simulink model "Scenario_2_v2"  (R2020b)
settings: Solver=ode1  StartTime=0.0  StopTime=10  FixedStep=Ts  MaxStep=Ts*2  MinStep=Ts/5  RelTol=1e-3
values from neighbouring files (symbols this model uses):
  c0 = c0_zeb    (= 6.57988e-09)    [Scenario_17_parameters_v2.m]    (also in Scenario_1_parameters_v2.m; Scenario_2_parameters_v2.m; Scenario_3_parameters_v2.m)
  c1 = c1_zeb    (= 9.15905e-09)    [Scenario_17_parameters_v2.m]    (also in Scenario_1_parameters_v2.m; Scenario_2_parameters_v2.m; Scenario_3_parameters_v2.m)
  fg = 50    [Scenario_17_parameters_v2.m]    (also in Scenario_1_parameters_v2.m; Scenario_2_parameters_v2.m; Scenario_3_parameters_v2.m)
  G1gen = 0.4692    [Scenario_17_parameters_v2.m]    (also in Scenario_1_parameters_v2.m = 0.1; Scenario_2_parameters_v2.m = 0.298581; Scenario_3_parameters_v2.m = 0.65)
  G2gen = 0.80    (= 0.8)    [Scenario_1_parameters_v2.m]    (also in Scenario_2_parameters_v2.m = 0.7; Scenario_3_parameters_v2.m = 0.4)
  G3gen = 0.85    [Scenario_1_parameters_v2.m]    (also in Scenario_2_parameters_v2.m = 0.9; Scenario_3_parameters_v2.m = 0.6)
  G4sgen = 0.8186    [Scenario_2_parameters_v2.m]
  G5gen = 0.75    [Scenario_17_parameters_v2.m]    (also in Scenario_1_parameters_v2.m = 0.8; Scenario_2_parameters_v2.m = 0.8; Scenario_3_parameters_v2.m = 0.705)
  G6gen = 0.90    (= 0.9)    [Scenario_17_parameters_v2.m]    (also in Scenario_1_parameters_v2.m; Scenario_2_parameters_v2.m = 0.81797; Scenario_3_parameters_v2.m = 0.45)
  G6sgen = 0.7    [Scenario_2_parameters_v2.m]
  G7gen = 0.20    (= 0.2)    [Scenario_17_parameters_v2.m]    (also in Scenario_1_parameters_v2.m = 0.5227; Scenario_2_parameters_v2.m = 0.5098; Scenario_3_parameters_v2.m = 0.4)
  Iovc = 1.2    [Scenario_17_parameters_v2.m]    (also in Scenario_1_parameters_v2.m; Scenario_2_parameters_v2.m; Scenario_3_parameters_v2.m)
  l0 = l0_zeb    (= 0.00368)    [Scenario_17_parameters_v2.m]    (also in Scenario_1_parameters_v2.m; Scenario_2_parameters_v2.m; Scenario_3_parameters_v2.m)
  l1 = l1_zeb    (= 0.00128)    [Scenario_17_parameters_v2.m]    (also in Scenario_1_parameters_v2.m; Scenario_2_parameters_v2.m; Scenario_3_parameters_v2.m)
  L3dem = 0.30    (= 0.3)    [Scenario_17_parameters_v2.m]    (also in Scenario_1_parameters_v2.m = 0.1; Scenario_2_parameters_v2.m = 0.1; Scenario_3_parameters_v2.m = 0.2)
  L4dem = 0.30    (= 0.3)    [Scenario_1_parameters_v2.m]    (also in Scenario_2_parameters_v2.m)
  L5dem = 0.25    [Scenario_17_parameters_v2.m]    (also in Scenario_1_parameters_v2.m = 0.35; Scenario_2_parameters_v2.m = 0.35; Scenario_3_parameters_v2.m = 0.1)
  L6dem = 0.15    [Scenario_1_parameters_v2.m]    (also in Scenario_2_parameters_v2.m; Scenario_3_parameters_v2.m = 0.1)
  L7dem = 0.10    (= 0.1)    [Scenario_1_parameters_v2.m]    (also in Scenario_2_parameters_v2.m; Scenario_3_parameters_v2.m = 0.2)
  Pr = Sr*PF    (= 1600500000)    [Scenario_17_parameters_v2.m]    (also in Scenario_1_parameters_v2.m = 1472500000; Scenario_2_parameters_v2.m = 1805000000; Scenario_3_parameters_v2.m = 12740000000)
  Qr = sqrt(Sr^2 - Pr^2)    [Scenario_17_parameters_v2.m]    (also in Scenario_1_parameters_v2.m; Scenario_2_parameters_v2.m; Scenario_3_parameters_v2.m)
  r0 = r0_zeb    (= 0.39362)    [Scenario_17_parameters_v2.m]    (also in Scenario_1_parameters_v2.m; Scenario_2_parameters_v2.m; Scenario_3_parameters_v2.m)
  r1 = r1_zeb    (= 0.06862)    [Scenario_17_parameters_v2.m]    (also in Scenario_1_parameters_v2.m; Scenario_2_parameters_v2.m; Scenario_3_parameters_v2.m)
  Rtpu = Xtpu/40    (= 0.0025)    [Scenario_17_parameters_v2.m]    (also in Scenario_1_parameters_v2.m = 0.00375; Scenario_2_parameters_v2.m = 0.00375; Scenario_3_parameters_v2.m)
  S1non = 700e6    (= 700000000)    [Scenario_17_parameters_v2.m]    (also in Scenario_1_parameters_v2.m = 400000000; Scenario_2_parameters_v2.m = 400000000; Scenario_3_parameters_v2.m = 1000000000)
  S2non = 300e6    (= 300000000)    [Scenario_1_parameters_v2.m]    (also in Scenario_2_parameters_v2.m; Scenario_3_parameters_v2.m = 3000000000)
  S3non = 200e6    (= 200000000)    [Scenario_1_parameters_v2.m]    (also in Scenario_2_parameters_v2.m; Scenario_3_parameters_v2.m = 1000000000)
  S4snon = 200e6    (= 200000000)    [Scenario_2_parameters_v2.m]
  S5non = 400e6    (= 400000000)    [Scenario_17_parameters_v2.m]    (also in Scenario_1_parameters_v2.m = 500000000; Scenario_2_parameters_v2.m = 500000000; Scenario_3_parameters_v2.m = 2000000000)
  S6non = 150e6    (= 150000000)    [Scenario_17_parameters_v2.m]    (also in Scenario_1_parameters_v2.m = 400000000; Scenario_2_parameters_v2.m = 400000000; Scenario_3_parameters_v2.m = 3000000000)
  S6snon = 200e6    (= 200000000)    [Scenario_2_parameters_v2.m]
  S7non = 1500e6    (= 1500000000)    [Scenario_17_parameters_v2.m]    (also in Scenario_1_parameters_v2.m = 200000000; Scenario_2_parameters_v2.m = 200000000; Scenario_3_parameters_v2.m = 4000000000)
  tonvsc = 0    [Scenario_17_parameters_v2.m]    (also in Scenario_1_parameters_v2.m; Scenario_2_parameters_v2.m; Scenario_3_parameters_v2.m = 0.0001)
  Ts = 50e-6    (= 5e-05)    [Scenario_17_parameters_v2.m]    (also in Scenario_1_parameters_v2.m = 0.0002; Scenario_2_parameters_v2.m = 2e-05; Scenario_3_parameters_v2.m = 0.0001)
  Vhv = 220e3    (= 220000)    [Scenario_17_parameters_v2.m]    (also in Scenario_1_parameters_v2.m; Scenario_2_parameters_v2.m; Scenario_3_parameters_v2.m)
  Vmv = 22e3    (= 22000)    [Scenario_17_parameters_v2.m]    (also in Scenario_1_parameters_v2.m; Scenario_2_parameters_v2.m; Scenario_3_parameters_v2.m)
  w_pll = 2*pi*80    (= 502.654824574)    [Scenario_17_parameters_v2.m]    (also in Scenario_1_parameters_v2.m; Scenario_2_parameters_v2.m; Scenario_3_parameters_v2.m)
  wc1 = wsw1/10    (= 848.230016469)    [Scenario_17_parameters_v2.m]    (also in Scenario_1_parameters_v2.m; Scenario_2_parameters_v2.m; Scenario_3_parameters_v2.m)
  wdc1 = wc1/10    (= 84.8230016469)    [Scenario_17_parameters_v2.m]    (also in Scenario_1_parameters_v2.m; Scenario_2_parameters_v2.m; Scenario_3_parameters_v2.m)
  wpq1 = wc1/10    (= 84.8230016469)    [Scenario_17_parameters_v2.m]    (also in Scenario_1_parameters_v2.m; Scenario_2_parameters_v2.m; Scenario_3_parameters_v2.m)
  wsw1 = ksw1*2*pi*fg    (= 8482.30016469)    [Scenario_17_parameters_v2.m]    (also in Scenario_1_parameters_v2.m; Scenario_2_parameters_v2.m; Scenario_3_parameters_v2.m)
  Xtpu = 0.10    (= 0.1)    [Scenario_17_parameters_v2.m]    (also in Scenario_1_parameters_v2.m = 0.15; Scenario_2_parameters_v2.m = 0.15; Scenario_3_parameters_v2.m)
undefined symbols (not defined in the file or in its folder): D11, Delta, Newton, Raphson
libraries: powerlib x214, simulink_extras x133, powerlib_meascontrol x102, pid_lib x48, simulink x32, eeTransforms x24, spsFirstOrderFilterLib x16, eePwmGeneratorTwoLevel x4
(part 1 of 19)
settings Model: Creator=User  LastModifiedBy=Usuario
settings SolverCC: InitialStep=Ts
settings DebuggingCC: UnconnectedInputMsg=none  UnconnectedOutputMsg=none  UnconnectedLineMsg=none

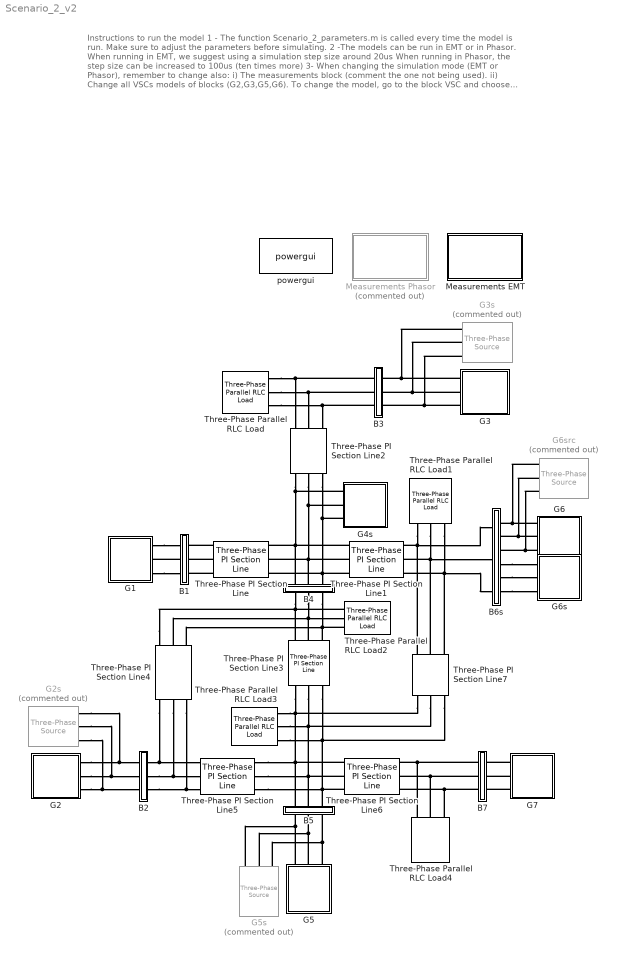
== system Scenario_2_v2 ==
  note: Instructions to run the model
      |
      | 1 - The function Scenario_2_parameters.m is called every time the model is run. Make sure to adjust the parameters before simulating.
      | 2 -The models can be run in EMT or in Phasor.
      | 	When running in EMT, we suggest using a simulation step size around 20us
      | 	When running in Phasor, the step size can be increased to 100us (ten times more)
      | 3- When changing the simulation mode (EMT or Phasor), remember to change also:
      | 	i) The measurements block (comment the one not being used).
      | 	ii) Change all VSCs models of blocks (G2,G3,G5,G6).
      | 	    To change the model, go to the block VSC and choose one model of droplist under the parameter 'VSC model'
      | 	    We recommend the model AVG model for EMT and the I-ref model for Phasor.
      | 4- The synchronous generators were initialized using power flow to have a near-flat initialization.
      |      As the VSCs are not standard blocks in Simulink, they are not considered in the power flow.
      |     To consider them, connect the voltage source in their place and run the power flow. Then, substitute by the VSCs.
  B1 : Subsystem
  B2 : Subsystem
  B3 : Subsystem
  B4 : Subsystem
  B5 : Subsystem
  B6s : Subsystem
  B7 : Subsystem
  G1 : Subsystem
      mask Display:
      | disp('SG')
      | %x = [0:0.001:1];
      | %y = 0.2*sin(10*x) + 0.5;
      | %plot(x,y)
  G2 : Subsystem
  G2s : powerlib/Electrical Sources/Three-Phase Source  Commented=on  InternalConnection=Yg  VoltagePhases=off  Voltage=(220000)*0.989022  PhaseAngle=-26.0473  Voltage_phases=[25e3 25e3 25e3]/sqrt(3)  PhaseAngles_phases=[0 -120 +120]  Frequency=fg  NonIdealSource=on  SpecifyImpedance=off  Resistance=Rtpu*(Vhv^2/S2non)  Inductance=Xtpu*(Vhv^2/S2non) * 1/(2*pi*fg)  ShortCircuitLevel=Svsc1  BaseVoltage=Vhv  XRratio=Xtpu/Rtpu  BusType=PQ  Pref=S2non*G2gen  Qref=50e6  Prefabc=[10e3, 10e3, 10e3]  Qrefabc=[0, 0, 0]  Qmin=-inf  Qmax=inf
  G3 : Subsystem
  G3s : powerlib/Electrical Sources/Three-Phase Source  Commented=on  InternalConnection=Yg  VoltagePhases=off  Voltage=(220000)*1.00116  PhaseAngle=-25.2337  Voltage_phases=[25e3 25e3 25e3]/sqrt(3)  PhaseAngles_phases=[0 -120 +120]  Frequency=fg  NonIdealSource=on  SpecifyImpedance=off  Resistance=Rtpu*(Vhv^2/S3non)  Inductance=Xtpu*(Vhv^2/S3non) * 1/(2*pi*fg)  ShortCircuitLevel=Svsc1  BaseVoltage=Vhv  XRratio=Xtpu/Rtpu  BusType=PQ  Pref=S3non*G3gen  Qref=50e6  Prefabc=[10e3, 10e3, 10e3]  Qrefabc=[0, 0, 0]  Qmin=-inf  Qmax=inf
  G4s : Subsystem
      mask Display: disp('SG')
  G5 : Subsystem
  G5s : powerlib/Electrical Sources/Three-Phase Source  Commented=on  InternalConnection=Yg  VoltagePhases=off  Voltage=(220000)*0.972267  PhaseAngle=-25.9849  Voltage_phases=[25e3 25e3 25e3]/sqrt(3)  PhaseAngles_phases=[0 -120 +120]  Frequency=fg  NonIdealSource=on  SpecifyImpedance=off  Resistance=Rtpu*(Vhv^2/S5non)  Inductance=Xtpu*(Vhv^2/S5non) * 1/(2*pi*fg)  ShortCircuitLevel=Svsc1  BaseVoltage=Vhv  XRratio=Xtpu/Rtpu  BusType=PQ  Pref=S5non*G5gen  Qref=50e6  Prefabc=[10e3, 10e3, 10e3]  Qrefabc=[0, 0, 0]  Qmin=-inf  Qmax=inf
  G6 : Subsystem
  G6s : Subsystem
      mask Display: disp('SG')
  G6src : powerlib/Electrical Sources/Three-Phase Source  Commented=on  InternalConnection=Yg  VoltagePhases=off  Voltage=(220000)*0.985009  PhaseAngle=-24.8902  Voltage_phases=[25e3 25e3 25e3]/sqrt(3)  PhaseAngles_phases=[0 -120 +120]  Frequency=fg  NonIdealSource=on  SpecifyImpedance=off  Resistance=Rtpu*(Vhv^2/S6non)  Inductance=Xtpu*(Vhv^2/S6non) * 1/(2*pi*fg)  ShortCircuitLevel=Svsc1  BaseVoltage=Vhv  XRratio=Xtpu/Rtpu  BusType=PQ  Pref=S6non*G6gen  Qref=50e6  Prefabc=[10e3, 10e3, 10e3]  Qrefabc=[0, 0, 0]  Qmin=-inf  Qmax=inf
  G7 : Subsystem
      mask Display:
      | disp('SG')
      | %x = [0:0.001:1];
      | %y = 0.2*sin(10*x) + 0.5;
      | %plot(x,y)
  Measurements EMT : Subsystem
  Measurements Phasor : Subsystem  Commented=on
  Three-Phase PI Section Line : powerlib/Elements/Three-Phase PI Section Line  LConnTagsString=a|b|c  RConnTagsString=A|B|C  Length=40  Frequency=fg  Resistances=[r1 r0]  Inductances="[l1  l0]"  Capacitances=[c1 c0]
  Three-Phase PI Section Line{1,4..5,7} (4 alike) : powerlib/Elements/Three-Phase PI Section Line  LConnTagsString=a|b|c  RConnTagsString=A|B|C  Length=20  Frequency=fg  Resistances=[r1 r0]  Inductances="[l1  l0]"  Capacitances=[c1 c0]
  Three-Phase PI Section Line2 : powerlib/Elements/Three-Phase PI Section Line  LConnTagsString=a|b|c  RConnTagsString=A|B|C  Length=10  Frequency=fg  Resistances=[r1 r0]  Inductances="[l1  l0]"  Capacitances=[c1 c0]
  Three-Phase PI Section Line3 : powerlib/Elements/Three-Phase PI Section Line  LConnTagsString=a|b|c  RConnTagsString=A|B|C  Length=10  Frequency=fg  Resistances=[r1 r0]  Inductances="[l1  l0]"  Capacitances=[c1 c0]
  Three-Phase PI Section Line6 : powerlib/Elements/Three-Phase PI Section Line  LConnTagsString=a|b|c  RConnTagsString=A|B|C  Length=30  Frequency=fg  Resistances=[r1 r0]  Inductances="[l1  l0]"  Capacitances=[c1 c0]
  Three-Phase Parallel RLC Load : powerlib/Elements/Three-Phase Parallel RLC Load  LConnTagsString=A|B|C  Configuration=Y (grounded)  NominalVoltage=Vhv  Vabc=[1e3 1e3 1e3]  Vabcp=[1e3 1e3 1e3]  NominalFrequency=fg  UnbalancedPower=off  ActivePower=Pr*L3dem  InductivePower=Qr*L3dem  CapacitivePower=0  Pabc=[10e3 9e3 11e3]  QLabc=[100 90 110]  QCabc=[100 90 110]  Pabcp=[10e3 9e3 11e3]  QLabcp=[100 90 110]  QCabcp=[100 90 110]  Measurements=None  LoadType=constant Z
  Three-Phase Parallel RLC Load1 : powerlib/Elements/Three-Phase Parallel RLC Load  LConnTagsString=A|B|C  Configuration=Y (grounded)  NominalVoltage=Vhv  Vabc=[1e3 1e3 1e3]  Vabcp=[1e3 1e3 1e3]  NominalFrequency=fg  UnbalancedPower=off  ActivePower=Pr*L6dem  InductivePower=Qr*L6dem  CapacitivePower=0  Pabc=[10e3 9e3 11e3]  QLabc=[100 90 110]  QCabc=[100 90 110]  Pabcp=[10e3 9e3 11e3]  QLabcp=[100 90 110]  QCabcp=[100 90 110]  Measurements=None  LoadType=constant Z
  Three-Phase Parallel RLC Load2 : powerlib/Elements/Three-Phase Parallel RLC Load  LConnTagsString=A|B|C  Configuration=Y (grounded)  NominalVoltage=Vhv  Vabc=[1e3 1e3 1e3]  Vabcp=[1e3 1e3 1e3]  NominalFrequency=fg  UnbalancedPower=off  ActivePower=Pr*L4dem  InductivePower=Qr*L4dem  CapacitivePower=0  Pabc=[10e3 9e3 11e3]  QLabc=[100 90 110]  QCabc=[100 90 110]  Pabcp=[10e3 9e3 11e3]  QLabcp=[100 90 110]  QCabcp=[100 90 110]  Measurements=None  LoadType=constant Z
  Three-Phase Parallel RLC Load3 : powerlib/Elements/Three-Phase Parallel RLC Load  LConnTagsString=A|B|C  Configuration=Y (grounded)  NominalVoltage=Vhv  Vabc=[1e3 1e3 1e3]  Vabcp=[1e3 1e3 1e3]  NominalFrequency=fg  UnbalancedPower=off  ActivePower=Pr*L5dem  InductivePower=Qr*L5dem  CapacitivePower=0  Pabc=[10e3 9e3 11e3]  QLabc=[100 90 110]  QCabc=[100 90 110]  Pabcp=[10e3 9e3 11e3]  QLabcp=[100 90 110]  QCabcp=[100 90 110]  Measurements=None  LoadType=constant Z
  Three-Phase Parallel RLC Load4 : powerlib/Elements/Three-Phase Parallel RLC Load  LConnTagsString=A|B|C  Configuration=Y (grounded)  NominalVoltage=Vhv  Vabc=[1e3 1e3 1e3]  Vabcp=[1e3 1e3 1e3]  NominalFrequency=fg  UnbalancedPower=off  ActivePower=Pr*L7dem  InductivePower=Qr*L7dem  CapacitivePower=0  Pabc=[10e3 9e3 11e3]  QLabc=[100 90 110]  QCabc=[100 90 110]  Pabcp=[10e3 9e3 11e3]  QLabcp=[100 90 110]  QCabcp=[100 90 110]  Measurements=None  LoadType=constant Z
  powergui : powerlib/powergui  Priority=1  SimulationMode=Discrete  SampleTime=Ts  frequency=fg  Iterations=50  frequencyindice=50  Pbase=100e6  ErrMax=0.0001  UnitsV=kV  UnitsW=MW  buscounter=0  FunctionMessages=off  echomessages=off  EnableUseOfTLC=off  CurrentSourceSwitches=off  DisableSnubberDevices=off  DisableRonSwitches=off  DisableVfSwitches=off  DisplayEquations=off  AutomaticDiscreteSolvers=off  SolverType=Tustin/Backward Euler (TBE)  Interpol=off  ExternalGateDelay=off  methode=off  Ts=100  x0status=blocks  SPID=on  SwTol=0  HookPort=off  NonlinearTolerance=1e-4  nMaxIteration=100  ContinueOnMaxIteration=off  RestoreLinks=warning  ResistiveCurrentMeasurement=off  Frange=[0:2:500]  Ylog=off  Xlog=on  ShowGrid=off  save=off  variable=ZData  structure=0  ZoomFFT=off  StartTime=0.0  cycles=1  DisplayStyle=1  fundamental=60  FreqAxis=off  MaxFrequency=1000  frequencyindicesteady=1  RmsSteady=2  display=off
  connections:
  Three-Phase PI Section Line/LConn1 -- B1/RConn1
  Three-Phase PI Section Line/LConn2 -- B1/RConn2
  Three-Phase PI Section Line/LConn3 -- B1/RConn3
  Three-Phase PI Section Line4/RConn1 -- B4/RConn1 -- Three-Phase PI Section Line3/RConn1 -- Three-Phase Parallel RLC Load2/LConn1
  Three-Phase Parallel RLC Load/LConn1 -- Three-Phase PI Section Line2/RConn1 -- B3/RConn1
  Three-Phase Parallel RLC Load/LConn2 -- B3/RConn2 -- Three-Phase PI Section Line2/RConn2
  Three-Phase Parallel RLC Load/LConn3 -- B3/RConn3 -- Three-Phase PI Section Line2/RConn3
  Three-Phase PI Section Line7/RConn1 -- Three-Phase Parallel RLC Load1/LConn1 -- B6s/LConn1 -- Three-Phase PI Section Line1/RConn1
  Three-Phase Parallel RLC Load1/LConn2 -- Three-Phase PI Section Line7/RConn2 -- B6s/LConn2 -- Three-Phase PI Section Line1/RConn2
  Three-Phase Parallel RLC Load1/LConn3 -- Three-Phase PI Section Line7/RConn3 -- B6s/LConn3 -- Three-Phase PI Section Line1/RConn3
  B5/RConn1 -- Three-Phase PI Section Line6/LConn1 -- Three-Phase Parallel RLC Load3/LConn1 -- Three-Phase PI Section Line3/LConn1 -- Three-Phase PI Section Line7/LConn1 -- Three-Phase PI Section Line5/RConn1
  B5/RConn2 -- Three-Phase PI Section Line6/LConn2 -- Three-Phase PI Section Line5/RConn2 -- Three-Phase Parallel RLC Load3/LConn2 -- Three-Phase PI Section Line3/LConn2 -- Three-Phase PI Section Line7/LConn2
  B5/RConn3 -- Three-Phase PI Section Line6/LConn3 -- Three-Phase Parallel RLC Load3/LConn3 -- Three-Phase PI Section Line3/LConn3 -- Three-Phase PI Section Line7/LConn3 -- Three-Phase PI Section Line5/RConn3
  B2/RConn1 -- Three-Phase PI Section Line5/LConn1 -- Three-Phase PI Section Line4/LConn1
  B2/RConn2 -- Three-Phase PI Section Line5/LConn2 -- Three-Phase PI Section Line4/LConn2
  B2/RConn3 -- Three-Phase PI Section Line4/LConn3 -- Three-Phase PI Section Line5/LConn3
  B7/RConn1 -- Three-Phase Parallel RLC Load4/LConn1 -- Three-Phase PI Section Line6/RConn1
  B7/RConn3 -- Three-Phase PI Section Line6/RConn3 -- Three-Phase Parallel RLC Load4/LConn3
  B7/RConn2 -- Three-Phase PI Section Line6/RConn2 -- Three-Phase Parallel RLC Load4/LConn2
  G7/RConn1 -- B7/LConn1
  G7/RConn2 -- B7/LConn2
  G7/RConn3 -- B7/LConn3
  Three-Phase PI Section Line2/LConn3 -- G4s/RConn3 -- B4/LConn3 -- Three-Phase PI Section Line/RConn3 -- Three-Phase PI Section Line1/LConn3
  Three-Phase PI Section Line1/LConn1 -- Three-Phase PI Section Line2/LConn1 -- G4s/RConn1 -- B4/LConn1 -- Three-Phase PI Section Line/RConn1
  Three-Phase PI Section Line1/LConn2 -- Three-Phase PI Section Line2/LConn2 -- G4s/RConn2 -- Three-Phase PI Section Line/RConn2 -- B4/LConn2
  B6s/RConn4 -- G6s/RConn1
  B6s/RConn5 -- G6s/RConn2
  B6s/RConn6 -- G6s/RConn3
  G5/RConn1 -- G5s/RConn1 -- B5/LConn1
  G5/RConn2 -- G5s/RConn2 -- B5/LConn2
  G5/RConn3 -- G5s/RConn3 -- B5/LConn3
  G2/RConn1 -- G2s/RConn1 -- B2/LConn1
  G2/RConn2 -- G2s/RConn2 -- B2/LConn2
  G2/RConn3 -- G2s/RConn3 -- B2/LConn3
  G3/RConn1 -- B3/LConn1 -- G3s/RConn1
  G3/RConn2 -- G3s/RConn2 -- B3/LConn2
  G3/RConn3 -- G3s/RConn3 -- B3/LConn3
  G6/RConn1 -- G6src/RConn1 -- B6s/RConn1
  G6/RConn2 -- G6src/RConn2 -- B6s/RConn2
  G6/RConn3 -- G6src/RConn3 -- B6s/RConn3
  G1/RConn3 -- B1/LConn3
  G1/RConn1 -- B1/LConn1
  B1/LConn2 -- G1/RConn2
  Three-Phase PI Section Line4/RConn2 -- Three-Phase Parallel RLC Load2/LConn2 -- B4/RConn2 -- Three-Phase PI Section Line3/RConn2
  Three-Phase PI Section Line4/RConn3 -- Three-Phase Parallel RLC Load2/LConn3 -- B4/RConn3 -- Three-Phase PI Section Line3/RConn3

== system Scenario_2_v2/B1 ==
  Current Measurement : powerlib/Measurements/Current Measurement  PhasorSimulation=off  OutputType=Complex  PSBequivalent=0
  Current Measurement1 : powerlib/Measurements/Current Measurement  PhasorSimulation=off  OutputType=Complex  PSBequivalent=0
  Current Measurement2 : powerlib/Measurements/Current Measurement  PhasorSimulation=off  OutputType=Complex  PSBequivalent=0
  Gain : Gain
  Gain1 : Gain
  Ground : powerlib/Elements/Ground  LConnTagsString=a
  Ground1 : powerlib/Elements/Ground  LConnTagsString=a
  Ground2 : powerlib/Elements/Ground  LConnTagsString=a
  Load Flow Bus : powerlib/Measurements/Load Flow Bus  LConnTagsString=a  Phases=single  Connectors=on one side  ID=B1  Vbase=Vhv  Vref=1  Vangle=0  VLF=0.9799  VLFb=1  VLFc=1  angleLF=-31.53  angleLFb=0  angleLFc=0
  Mux : Mux  Inputs=3
  Mux1 : Mux  Inputs=3
  Voltage Measurement : powerlib/Measurements/Voltage Measurement  PhasorSimulation=off  OutputType=Complex  PSBequivalent=0
  Voltage Measurement1 : powerlib/Measurements/Voltage Measurement  PhasorSimulation=off  OutputType=Complex  PSBequivalent=0
  Voltage Measurement2 : powerlib/Measurements/Voltage Measurement  PhasorSimulation=off  OutputType=Complex  PSBequivalent=0
  A : PMIOPort  Side=Left
  B : PMIOPort  Port=2  Side=Left
  C : PMIOPort  Port=3  Side=Left
  a : PMIOPort  Port=4  Side=Right
  b : PMIOPort  Port=5  Side=Right
  c : PMIOPort  Port=6  Side=Right
  tag scope: Ig1=global, Vg1=global
  wires:
  Voltage Measurement2/1 -> Mux/3
  Voltage Measurement1/1 -> Mux/2
  Voltage Measurement/1 -> Mux/1
  Current Measurement/1 -> Mux1/1
  Current Measurement1/1 -> Mux1/2
  Current Measurement2/1 -> Mux1/3
  Mux/1 -> Gain/1
  Gain/1 -> [Vg1]
  Mux1/1 -> Gain1/1
  Gain1/1 -> [Ig1]
  connections:
  Current Measurement/RConn1 -- a/RConn1
  Current Measurement1/LConn1 -- Voltage Measurement1/LConn1 -- B/RConn1
  Current Measurement2/LConn1 -- Voltage Measurement2/LConn1 -- C/RConn1
  Current Measurement/LConn1 -- Voltage Measurement/LConn1 -- Load Flow Bus/LConn1 -- A/RConn1
  Current Measurement1/RConn1 -- b/RConn1
  Current Measurement2/RConn1 -- c/RConn1
  Ground/LConn1 -- Voltage Measurement/LConn2
  Ground1/LConn1 -- Voltage Measurement1/LConn2
  Ground2/LConn1 -- Voltage Measurement2/LConn2

== system Scenario_2_v2/B2 ==
  Current Measurement : powerlib/Measurements/Current Measurement  PhasorSimulation=off  OutputType=Complex  PSBequivalent=0
  Current Measurement1 : powerlib/Measurements/Current Measurement  PhasorSimulation=off  OutputType=Complex  PSBequivalent=0
  Current Measurement2 : powerlib/Measurements/Current Measurement  PhasorSimulation=off  OutputType=Complex  PSBequivalent=0
  Gain : Gain
  Gain1 : Gain
  Ground : powerlib/Elements/Ground  LConnTagsString=a
  Ground1 : powerlib/Elements/Ground  LConnTagsString=a
  Ground2 : powerlib/Elements/Ground  LConnTagsString=a
  Load Flow Bus3 : powerlib/Measurements/Load Flow Bus  LConnTagsString=a  Phases=single  Connectors=on one side  ID=B2  Vbase=Vhv  Vref=1  Vangle=0  VLF=0.954  VLFb=1  VLFc=1  angleLF=-32.4  angleLFb=0  angleLFc=0
  Mux : Mux  Inputs=3
  Mux1 : Mux  Inputs=3
  Voltage Measurement : powerlib/Measurements/Voltage Measurement  PhasorSimulation=off  OutputType=Complex  PSBequivalent=0
  Voltage Measurement1 : powerlib/Measurements/Voltage Measurement  PhasorSimulation=off  OutputType=Complex  PSBequivalent=0
  Voltage Measurement2 : powerlib/Measurements/Voltage Measurement  PhasorSimulation=off  OutputType=Complex  PSBequivalent=0
  A : PMIOPort  Side=Left
  B : PMIOPort  Port=2  Side=Left
  C : PMIOPort  Port=3  Side=Left
  a : PMIOPort  Port=4  Side=Right
  b : PMIOPort  Port=5  Side=Right
  c : PMIOPort  Port=6  Side=Right
  tag scope: Ig2=global, Vg2=global
  wires:
  Voltage Measurement2/1 -> Mux/3
  Voltage Measurement1/1 -> Mux/2
  Voltage Measurement/1 -> Mux/1
  Current Measurement/1 -> Mux1/1
  Current Measurement1/1 -> Mux1/2
  Current Measurement2/1 -> Mux1/3
  Mux/1 -> Gain/1
  Gain/1 -> [Vg2]
  Mux1/1 -> Gain1/1
  Gain1/1 -> [Ig2]
  connections:
  Current Measurement/RConn1 -- a/RConn1
  B/RConn1 -- Current Measurement1/LConn1 -- Voltage Measurement1/LConn1
  C/RConn1 -- Current Measurement2/LConn1 -- Voltage Measurement2/LConn1
  Voltage Measurement/LConn1 -- Load Flow Bus3/LConn1 -- A/RConn1 -- Current Measurement/LConn1
  Current Measurement1/RConn1 -- b/RConn1
  Current Measurement2/RConn1 -- c/RConn1
  Ground/LConn1 -- Voltage Measurement/LConn2
  Ground1/LConn1 -- Voltage Measurement1/LConn2
  Ground2/LConn1 -- Voltage Measurement2/LConn2

== system Scenario_2_v2/B3 ==
  Current Measurement : powerlib/Measurements/Current Measurement  PhasorSimulation=off  OutputType=Complex  PSBequivalent=0
  Current Measurement1 : powerlib/Measurements/Current Measurement  PhasorSimulation=off  OutputType=Complex  PSBequivalent=0
  Current Measurement2 : powerlib/Measurements/Current Measurement  PhasorSimulation=off  OutputType=Complex  PSBequivalent=0
  Gain : Gain
  Gain1 : Gain
  Ground : powerlib/Elements/Ground  LConnTagsString=a
  Ground1 : powerlib/Elements/Ground  LConnTagsString=a
  Ground2 : powerlib/Elements/Ground  LConnTagsString=a
  Load Flow Bus1 : powerlib/Measurements/Load Flow Bus  LConnTagsString=a  Phases=single  Connectors=on one side  ID=B3  Vbase=Vhv  Vref=1  Vangle=0  VLF=0.948  VLFb=1  VLFc=1  angleLF=-33.35  angleLFb=0  angleLFc=0
  Mux : Mux  Inputs=3
  Mux1 : Mux  Inputs=3
  Voltage Measurement : powerlib/Measurements/Voltage Measurement  PhasorSimulation=off  OutputType=Complex  PSBequivalent=0
  Voltage Measurement1 : powerlib/Measurements/Voltage Measurement  PhasorSimulation=off  OutputType=Complex  PSBequivalent=0
  Voltage Measurement2 : powerlib/Measurements/Voltage Measurement  PhasorSimulation=off  OutputType=Complex  PSBequivalent=0
  A : PMIOPort  Side=Left
  B : PMIOPort  Port=2  Side=Left
  C : PMIOPort  Port=3  Side=Left
  a : PMIOPort  Port=4  Side=Right
  b : PMIOPort  Port=5  Side=Right
  c : PMIOPort  Port=6  Side=Right
  tag scope: Ig3=global, Vg3=global
  wires:
  Voltage Measurement2/1 -> Mux/3
  Voltage Measurement1/1 -> Mux/2
  Voltage Measurement/1 -> Mux/1
  Current Measurement/1 -> Mux1/1
  Current Measurement1/1 -> Mux1/2
  Current Measurement2/1 -> Mux1/3
  Mux/1 -> Gain/1
  Gain/1 -> [Vg3]
  Mux1/1 -> Gain1/1
  Gain1/1 -> [Ig3]
  connections:
  Current Measurement/RConn1 -- a/RConn1
  B/RConn1 -- Current Measurement1/LConn1 -- Voltage Measurement1/LConn1
  C/RConn1 -- Current Measurement2/LConn1 -- Voltage Measurement2/LConn1
  Voltage Measurement/LConn1 -- Load Flow Bus1/LConn1 -- A/RConn1 -- Current Measurement/LConn1
  Current Measurement1/RConn1 -- b/RConn1
  Current Measurement2/RConn1 -- c/RConn1
  Ground/LConn1 -- Voltage Measurement/LConn2
  Ground1/LConn1 -- Voltage Measurement1/LConn2
  Ground2/LConn1 -- Voltage Measurement2/LConn2

== system Scenario_2_v2/B4 ==
  Current Measurement : powerlib/Measurements/Current Measurement  PhasorSimulation=off  OutputType=Complex  PSBequivalent=0
  Current Measurement1 : powerlib/Measurements/Current Measurement  PhasorSimulation=off  OutputType=Complex  PSBequivalent=0
  Current Measurement2 : powerlib/Measurements/Current Measurement  PhasorSimulation=off  OutputType=Complex  PSBequivalent=0
  Gain : Gain
  Gain1 : Gain
  Ground : powerlib/Elements/Ground  LConnTagsString=a
  Ground1 : powerlib/Elements/Ground  LConnTagsString=a
  Ground2 : powerlib/Elements/Ground  LConnTagsString=a
  Load Flow Bus2 : powerlib/Measurements/Load Flow Bus  LConnTagsString=a  Phases=single  Connectors=on one side  ID=B4  Vbase=Vhv  Vref=1  Vangle=0  VLF=0.948  VLFb=1  VLFc=1  angleLF=-33.45  angleLFb=0  angleLFc=0
  Mux : Mux  Inputs=3
  Mux1 : Mux  Inputs=3
  Voltage Measurement : powerlib/Measurements/Voltage Measurement  PhasorSimulation=off  OutputType=Complex  PSBequivalent=0
  Voltage Measurement1 : powerlib/Measurements/Voltage Measurement  PhasorSimulation=off  OutputType=Complex  PSBequivalent=0
  Voltage Measurement2 : powerlib/Measurements/Voltage Measurement  PhasorSimulation=off  OutputType=Complex  PSBequivalent=0
  A : PMIOPort  Side=Left
  B : PMIOPort  Port=2  Side=Left
  C : PMIOPort  Port=3  Side=Left
  a : PMIOPort  Port=4  Side=Right
  b : PMIOPort  Port=5  Side=Right
  c : PMIOPort  Port=6  Side=Right
  tag scope: Ig4=global, Vg4=global
  wires:
  Voltage Measurement2/1 -> Mux/3
  Voltage Measurement1/1 -> Mux/2
  Voltage Measurement/1 -> Mux/1
  Current Measurement/1 -> Mux1/1
  Current Measurement1/1 -> Mux1/2
  Current Measurement2/1 -> Mux1/3
  Mux/1 -> Gain/1
  Gain/1 -> [Vg4]
  Mux1/1 -> Gain1/1
  Gain1/1 -> [Ig4]
  connections:
  Current Measurement/RConn1 -- a/RConn1
  B/RConn1 -- Current Measurement1/LConn1 -- Voltage Measurement1/LConn1
  C/RConn1 -- Current Measurement2/LConn1 -- Voltage Measurement2/LConn1
  Voltage Measurement/LConn1 -- Load Flow Bus2/LConn1 -- A/RConn1 -- Current Measurement/LConn1
  Current Measurement1/RConn1 -- b/RConn1
  Current Measurement2/RConn1 -- c/RConn1
  Ground/LConn1 -- Voltage Measurement/LConn2
  Ground1/LConn1 -- Voltage Measurement1/LConn2
  Ground2/LConn1 -- Voltage Measurement2/LConn2

== system Scenario_2_v2/B5 ==
  Current Measurement : powerlib/Measurements/Current Measurement  PhasorSimulation=off  OutputType=Complex  PSBequivalent=0
  Current Measurement1 : powerlib/Measurements/Current Measurement  PhasorSimulation=off  OutputType=Complex  PSBequivalent=0
  Current Measurement2 : powerlib/Measurements/Current Measurement  PhasorSimulation=off  OutputType=Complex  PSBequivalent=0
  Gain : Gain
  Gain1 : Gain
  Ground : powerlib/Elements/Ground  LConnTagsString=a
  Ground1 : powerlib/Elements/Ground  LConnTagsString=a
  Ground2 : powerlib/Elements/Ground  LConnTagsString=a
  Load Flow Bus4 : powerlib/Measurements/Load Flow Bus  LConnTagsString=a  Phases=single  Connectors=on one side  ID=B5  Vbase=Vhv  Vref=1  Vangle=0  VLF=0.9449  VLFb=1  VLFc=1  angleLF=-33.47  angleLFb=0  angleLFc=0
  Mux : Mux  Inputs=3
  Mux1 : Mux  Inputs=3
  Voltage Measurement : powerlib/Measurements/Voltage Measurement  PhasorSimulation=off  OutputType=Complex  PSBequivalent=0
  Voltage Measurement1 : powerlib/Measurements/Voltage Measurement  PhasorSimulation=off  OutputType=Complex  PSBequivalent=0
  Voltage Measurement2 : powerlib/Measurements/Voltage Measurement  PhasorSimulation=off  OutputType=Complex  PSBequivalent=0
  A : PMIOPort  Side=Left
  B : PMIOPort  Port=2  Side=Left
  C : PMIOPort  Port=3  Side=Left
  a : PMIOPort  Port=4  Side=Right
  b : PMIOPort  Port=5  Side=Right
  c : PMIOPort  Port=6  Side=Right
  tag scope: Ig5=global, Vg5=global
  wires:
  Voltage Measurement2/1 -> Mux/3
  Voltage Measurement1/1 -> Mux/2
  Voltage Measurement/1 -> Mux/1
  Current Measurement/1 -> Mux1/1
  Current Measurement1/1 -> Mux1/2
  Current Measurement2/1 -> Mux1/3
  Mux/1 -> Gain/1
  Gain/1 -> [Vg5]
  Mux1/1 -> Gain1/1
  Gain1/1 -> [Ig5]
  connections:
  Current Measurement/RConn1 -- a/RConn1
  B/RConn1 -- Current Measurement1/LConn1 -- Voltage Measurement1/LConn1
  C/RConn1 -- Current Measurement2/LConn1 -- Voltage Measurement2/LConn1
  Voltage Measurement/LConn1 -- Load Flow Bus4/LConn1 -- A/RConn1 -- Current Measurement/LConn1
  Current Measurement1/RConn1 -- b/RConn1
  Current Measurement2/RConn1 -- c/RConn1
  Ground/LConn1 -- Voltage Measurement/LConn2
  Ground1/LConn1 -- Voltage Measurement1/LConn2
  Ground2/LConn1 -- Voltage Measurement2/LConn2

== system Scenario_2_v2/B6s ==
  note: -1 gain is used to keep the convention (positive current coming from the generators to the grid)
  Current Measurement{,1..5} (6 alike) : powerlib/Measurements/Current Measurement  PhasorSimulation=off  OutputType=Complex  PSBequivalent=0
  Gain : Gain  Gain=-1
  Gain1 : Gain  Gain=-1
  Ground : powerlib/Elements/Ground  LConnTagsString=a
  Ground1 : powerlib/Elements/Ground  LConnTagsString=a
  Ground2 : powerlib/Elements/Ground  LConnTagsString=a
  Load Flow Bus6 : powerlib/Measurements/Load Flow Bus  LConnTagsString=a  Phases=single  Connectors=on one side  ID=B6  Vbase=Vhv  Vref=1  Vangle=0  VLF=0.954  VLFb=1  VLFc=1  angleLF=-32.28  angleLFb=0  angleLFc=0
  Mux : Mux  Inputs=3
  Mux1 : Mux  Inputs=3
  Mux2 : Mux  Inputs=3
  Voltage Measurement1 : powerlib/Measurements/Voltage Measurement  PhasorSimulation=off  OutputType=Complex  PSBequivalent=0
  Voltage Measurement2 : powerlib/Measurements/Voltage Measurement  PhasorSimulation=off  OutputType=Complex  PSBequivalent=0
  Voltage Measurement3 : powerlib/Measurements/Voltage Measurement  PhasorSimulation=off  OutputType=Complex  PSBequivalent=0
  A : PMIOPort  Side=Left
  B : PMIOPort  Port=2  Side=Left
  C : PMIOPort  Port=3  Side=Left
  a1 : PMIOPort  Port=4  Side=Right
  b1 : PMIOPort  Port=5  Side=Right
  c1 : PMIOPort  Port=6  Side=Right
  a2 : PMIOPort  Port=7  Side=Right
  b2 : PMIOPort  Port=8  Side=Right
  c2 : PMIOPort  Port=9  Side=Right
  tag scope: Ig6pv=global, Ig6s=global, Vg6=global
  wires:
  Voltage Measurement2/1 -> Mux/3
  Voltage Measurement3/1 -> Mux/2
  Voltage Measurement1/1 -> Mux/1
  Mux/1 -> [Vg6]
  Current Measurement/1 -> Mux1/1
  Current Measurement1/1 -> Mux1/2
  Current Measurement2/1 -> Mux1/3
  Current Measurement3/1 -> Mux2/1
  Current Measurement4/1 -> Mux2/2
  Current Measurement5/1 -> Mux2/3
  Mux1/1 -> Gain/1
  Gain/1 -> [Ig6pv]
  Mux2/1 -> Gain1/1
  Gain1/1 -> [Ig6s]
  connections:
  Current Measurement/RConn1 -- a1/RConn1
  Current Measurement4/LConn1 -- Current Measurement1/LConn1 -- B/RConn1 -- Voltage Measurement3/LConn1
  Current Measurement5/LConn1 -- Current Measurement2/LConn1 -- C/RConn1 -- Voltage Measurement2/LConn1
  Current Measurement3/LConn1 -- Current Measurement/LConn1 -- Load Flow Bus6/LConn1 -- A/RConn1 -- Voltage Measurement1/LConn1
  Current Measurement1/RConn1 -- b1/RConn1
  Current Measurement2/RConn1 -- c1/RConn1
  Current Measurement3/RConn1 -- a2/RConn1
  Current Measurement4/RConn1 -- b2/RConn1
  Current Measurement5/RConn1 -- c2/RConn1
  Ground/LConn1 -- Voltage Measurement1/LConn2
  Ground1/LConn1 -- Voltage Measurement2/LConn2
  Ground2/LConn1 -- Voltage Measurement3/LConn2

== system Scenario_2_v2/B7 ==
  Current Measurement : powerlib/Measurements/Current Measurement  PhasorSimulation=off  OutputType=Complex  PSBequivalent=0
  Current Measurement1 : powerlib/Measurements/Current Measurement  PhasorSimulation=off  OutputType=Complex  PSBequivalent=0
  Current Measurement2 : powerlib/Measurements/Current Measurement  PhasorSimulation=off  OutputType=Complex  PSBequivalent=0
  Gain : Gain
  Gain1 : Gain
  Ground : powerlib/Elements/Ground  LConnTagsString=a
  Ground1 : powerlib/Elements/Ground  LConnTagsString=a
  Ground2 : powerlib/Elements/Ground  LConnTagsString=a
  Load Flow Bus5 : powerlib/Measurements/Load Flow Bus  LConnTagsString=a  Phases=single  Connectors=on one side  ID=B7  Vbase=Vhv  Vref=1  Vangle=0  VLF=0.9512  VLFb=1  VLFc=1  angleLF=-34.65  angleLFb=0  angleLFc=0
  Mux : Mux  Inputs=3
  Mux1 : Mux  Inputs=3
  Voltage Measurement : powerlib/Measurements/Voltage Measurement  PhasorSimulation=off  OutputType=Complex  PSBequivalent=0
  Voltage Measurement1 : powerlib/Measurements/Voltage Measurement  PhasorSimulation=off  OutputType=Complex  PSBequivalent=0
  Voltage Measurement2 : powerlib/Measurements/Voltage Measurement  PhasorSimulation=off  OutputType=Complex  PSBequivalent=0
  A : PMIOPort  Side=Left
  B : PMIOPort  Port=2  Side=Left
  C : PMIOPort  Port=3  Side=Left
  a : PMIOPort  Port=4  Side=Right
  b : PMIOPort  Port=5  Side=Right
  c : PMIOPort  Port=6  Side=Right
  tag scope: Ig7=global, Vg7=global
  wires:
  Voltage Measurement2/1 -> Mux/3
  Voltage Measurement1/1 -> Mux/2
  Voltage Measurement/1 -> Mux/1
  Current Measurement/1 -> Mux1/1
  Current Measurement1/1 -> Mux1/2
  Current Measurement2/1 -> Mux1/3
  Mux/1 -> Gain/1
  Gain/1 -> [Vg7]
  Mux1/1 -> Gain1/1
  Gain1/1 -> [Ig7]
  connections:
  Current Measurement/RConn1 -- a/RConn1
  B/RConn1 -- Current Measurement1/LConn1 -- Voltage Measurement1/LConn1
  C/RConn1 -- Current Measurement2/LConn1 -- Voltage Measurement2/LConn1
  Voltage Measurement/LConn1 -- Load Flow Bus5/LConn1 -- A/RConn1 -- Current Measurement/LConn1
  Current Measurement1/RConn1 -- b/RConn1
  Current Measurement2/RConn1 -- c/RConn1
  Ground/LConn1 -- Voltage Measurement/LConn2
  Ground1/LConn1 -- Voltage Measurement1/LConn2
  Ground2/LConn1 -- Voltage Measurement2/LConn2

== system Scenario_2_v2/G1 ==
  note: Synchronous Machine Model according to ENTSO-E
  note: Nomenclature (according to IEEE Std 421.1-2007):
      | Efd = Exciter output voltage (generator field voltage)
      | Ifd = Exciter output current (generator field current)
      | Vf = Excitation system stabilizer signal
      | Vfe = Signal proportional to exciter field current
      | Vl = Limiters and protective elements feedback
      | Vr = Regulator output
      | Vs = Power System Stabilizer (PSS) output
      | Vsi = Power System Stabilizer (PSS) inputs (shaft speed, frequency, generator electric power, and others
      | Vt = Generator terminal voltage
      | It = Generator terminal current
      | Vref = Voltage regulator reference signal
      | Vc = terminal voltage transducer output
  Bus Selector : BusSelector  OutputSignals=dw,w,vq,vd,iq,id,Peo,Te,delta
  Constant : Constant  Value=G1gen
  Exciter System : Subsystem
  Real-Imag to Complex : RealImagToComplex
  Real-Imag to Complex1 : RealImagToComplex
  Ref voltage (p.u) : Constant  Value=1.0
  Snubber : powerlib/Elements/Three-Phase Parallel RLC Load  LConnTagsString=A|B|C  Configuration=Y (grounded)  NominalVoltage=Vmv  Vabc=[1e3 1e3 1e3]  Vabcp=[1e3 1e3 1e3]  NominalFrequency=fg  UnbalancedPower=off  ActivePower=S1non*0.03  InductivePower=0  CapacitivePower=0  Pabc=[10e3 9e3 11e3]  QLabc=[100 90 110]  QCabc=[100 90 110]  Pabcp=[10e3 9e3 11e3]  QLabcp=[100 90 110]  QCabcp=[100 90 110]  Measurements=None  LoadType=constant Z
  Speed Governor : Subsystem  mask{R=0.05, T1=0.5, T2=3, T3=10, Dt=0, Vmin=0, Vmax=10, P0=G1gen}
      mask prompts: R "Controller droop (R)"; T1 "Governor time constant (T1)(sec)"; T2 "Turbine derivative time constant (T2)(sec)"; T3 "Turbine delay time constant (T3)(sec)"; Dt "Frictional losses factor (Dt)"; Vmin "Minimum gate limit (Vmin)(p.u)"; Vmax "Maximum gate limit (Vmax)(p.u)"; P0 "Initial power (p.u)"
      mask Display:
      | disp('TGOV')
      | 
      | port_label('input',1,'Pref')
      | port_label('input',2,'dw')
      | 
      | port_label('output',1,'Pm')
  Synchronous Machine pu Standard : powerlib/Machines/Synchronous Machine pu Standard  PresetModel=No  MechanicalLoad=Mechanical power Pm  ShowDetailedParameters=on  RotorType=Salient-pole  Units=per unit standard parameters  MeasurementBus=on  NominalParameters=[S1non Vmv fg]  Reactances1=[ 1.81, 0.3, 0.23, 1.76, 0.65, 0.25, 0.15 ]  Reactances2=[1.25 0.333 0.292 1.0 0.292 0.15]  dAxisTimeConstants=Open-circuit  qAxisTimeConstants=Open-circuit  TimeConstants1="[5  0.002  0.002]"  TimeConstants2=[ 8.0, 0.03, 1.0, 0.07 ]  TimeConstants3="[  4.49  0.0681  0.0513  ]"  TimeConstants4=[ 8.0, 0.03, 0.3371, 0.0295 ]  TimeConstants5=[ 1.01, 0.053, 0.1 ]  TimeConstants6=[ 1.3201, 0.023, 1.0, 0.07 ]  TimeConstants7=[0.012 0.003 0.003]  TimeConstants8=[ 1.3201, 0.0231, 0.3371, 0.0295 ]  StatorResistance=0.01  Mechanical=[5 0 2]  PolePairs=20  InitialConditions=[0 -76.1866 0.357288 0.357288 0.357288 -33.6834 -153.683 86.3166 1.30275]  SetSaturation=off  Saturation=[0.6404,0.7127,0.8441,0.9214,0.9956,1.082,1.19,1.316,1.457;0.7,0.7698,0.8872,0.9466,0.9969,1.046,1.1,1.151,1.201]  LoadFlowParameters=[4 269720000 0 0 60000000]  TsPowergui=0  TsBlock=-1  IterativeModel=Trapezoidal non iterative  IterativeDiscreteModel=Trapezoidal non iterative  BusType=swing  Pref=0  Qref=0  Qmin=-inf  Qmax=inf  PLF=0  QLF=0
  Three-Phase Transformer (Two Windings) : powerlib/Elements/Three-Phase Transformer (Two Windings)  Winding1Connection=Delta (D11)  Winding2Connection=Yg  CoreType=Three single-phase transformers  SetSaturation=off  Hysteresis=off  DataFile='hysteresis'  SetInitialFlux=off  Measurements=None  UNITS=pu  NominalPower=[S1non , fg ]  Winding1=[Vmv 0.00125 0.05]  Winding2=[Vhv 0.00125 0.05]  Rm=5000  Lm=5000  L0=0.5  Saturation=[ 0,0 ; 0.0024,1.2 ; 1.0,1.52 ]  InitialFluxes=[ 0.8 , -0.8 , 0.7 ]  BreakLoop=off  DiscreteSolver=Trapezoidal iterative  DataType=off  TransfoNumber=1
  A : PMIOPort  Side=Right
  B : PMIOPort  Port=2  Side=Right
  C : PMIOPort  Port=3  Side=Right
  tag scope: Pe1=global, Te1=global, wm1=global
  wires:
  Bus Selector/1 -> Speed Governor/2(dw), Exciter System/1(<dw>)  "<dw>"
  Bus Selector/4 -> Real-Imag to Complex/2  "<vd>"
  Bus Selector/3 -> Real-Imag to Complex/1  "<vq>"
  Bus Selector/5 -> Real-Imag to Complex1/1  "<iq>"
  Bus Selector/6 -> Real-Imag to Complex1/2  "<id>"
  Real-Imag to Complex/1 -> Exciter System/3(Vt)
  Real-Imag to Complex1/1 -> Exciter System/4(It)
  Bus Selector/8 -> [Te1]  "<Te>"
  Speed Governor/1(Pm) -> Synchronous Machine pu Standard/1
  Exciter System/1(Efd) -> Synchronous Machine pu Standard/2
  Synchronous Machine pu Standard/1 -> Bus Selector/1
  Constant/1 -> Speed Governor/1(RefL)
  Bus Selector/2 -> [wm1]  "<w>"
  Bus Selector/7 -> [Pe1], Exciter System/5(<Peo>)  "<Peo>"
  Ref voltage (p.u)/1 -> Exciter System/2(Vref)
  connections:
  Synchronous Machine pu Standard/RConn1 -- Three-Phase Transformer (Two Windings)/LConn1 -- Snubber/LConn1
  Synchronous Machine pu Standard/RConn3 -- Three-Phase Transformer (Two Windings)/LConn3 -- Snubber/LConn3
  Synchronous Machine pu Standard/RConn2 -- Three-Phase Transformer (Two Windings)/LConn2 -- Snubber/LConn2
  Three-Phase Transformer (Two Windings)/RConn1 -- A/RConn1
  Three-Phase Transformer (Two Windings)/RConn2 -- B/RConn1
  Three-Phase Transformer (Two Windings)/RConn3 -- C/RConn1
